simulink model "led_flash"  (R2023b)
settings: Solver=FixedStepAuto  StartTime=0.0  StopTime=999  RelTol=1e-3  EnableMultiTasking=on
libraries: mbedblockslib x11, raspberrypiIMUsensorslib x1, eeQuadratureDecoder x1
settings Model: ExtModeTrigDuration=10  Creator=Aidan  LastModifiedBy=Aidan
settings SolverCC: AutoInsertRateTranBlk=on
settings OptimizationCC: EnhancedBackFolding=on  PassReuseOutputArgsAs=Individual arguments  ZeroExternalMemoryAtStartup=off  ZeroInternalMemoryAtStartup=off  MaxStackSize=64  OptimizeBlockOrder=speed  DifferentSizesBufferReuse=on  OptimizationCustomize=off  EfficientTunableParamExpr=on
settings DebuggingCC: ParameterTunabilityLossMsg=error
settings HardwareCC: ProdBitPerPointer=32  ProdBitPerSizeT=32  ProdBitPerPtrDiffT=32  ProdLargestAtomicInteger=Long  ProdLargestAtomicFloat=Double  ProdWordSize=32  ProdLongLongMode=on  ProdHWDeviceType=ARM Compatible->ARM Cortex  UseEmbeddedCoderFeatures=off
settings SFSimCC: MATLABDynamicMemAlloc=off
settings RTWCC: Description=Embedded Coder  SystemTargetFile=ert.tlc  HardwareBoard=STM32 Nucleo F746ZG  TemplateMakefile=ert_default_tmf  Toolchain=GNU Tools for ARM Embedded Processors
settings CodeAppCC: ForceParamTrailComments=on  IgnoreCustomStorageClasses=off  OperatorAnnotations=on  SimulinkDataObjDesc=on  SFDataObjDesc=on  InsertBlockDesc=on
settings ERTTargetCC: SupportNonInlinedSFcns=on  ExtModeTransport=3  ExtModeStaticAlloc=on  ExtModeStaticAllocSize=2000  ExtModeMexFile=ext_xcp  ExtModeIntrfLevel=Level2 - Open

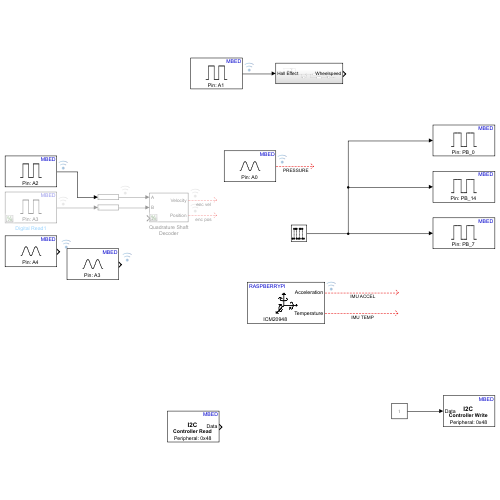
[thumbnail: Simulink's stored preview of the top-level diagram]
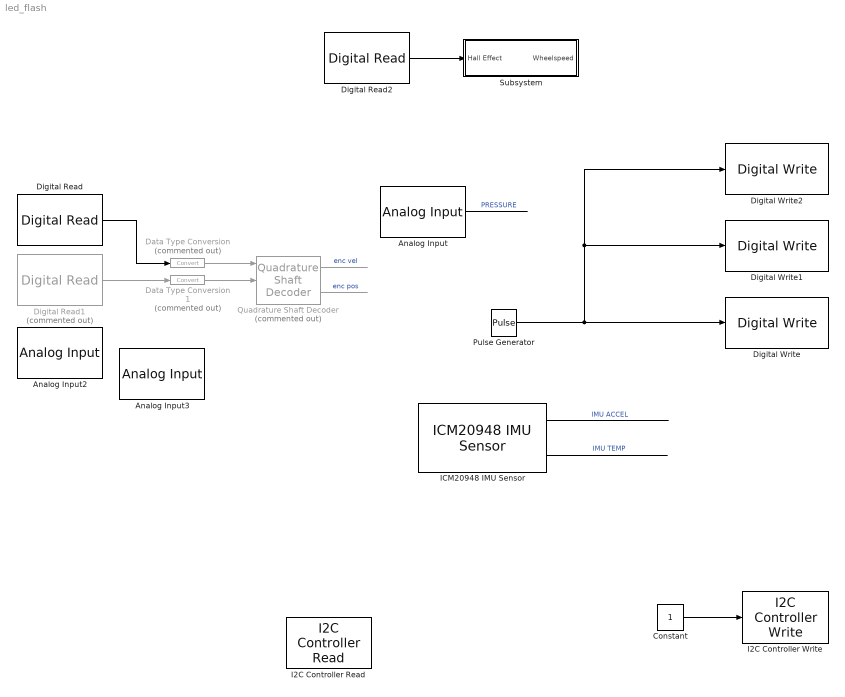
== system led_flash ==
  Analog Input : mbedblockslib/Analog Input  Pin=A0  ReadResultsOnly=off  ConversionTriggerSource=Software  ExternalTriggerType=uint32( 0 )  OutputDataType=double  EnableConversionCompleteNotify=off  EnableOuputStatus=off  SampleTime=-1
      settings: LibrarySourceBlock=stmnucleorootlib/Common/Analog Input
  Analog Input2 : mbedblockslib/Analog Input  Pin=A4  ReadResultsOnly=off  ConversionTriggerSource=Software  ExternalTriggerType=uint32( 0 )  OutputDataType=double  EnableConversionCompleteNotify=off  EnableOuputStatus=off  SampleTime=-1
      settings: LibrarySourceBlock=stmnucleorootlib/Common/Analog Input
  Analog Input3 : mbedblockslib/Analog Input  Pin=A3  ReadResultsOnly=off  ConversionTriggerSource=Software  ExternalTriggerType=uint32( 0 )  OutputDataType=double  EnableConversionCompleteNotify=off  EnableOuputStatus=off  SampleTime=-1
      settings: LibrarySourceBlock=stmnucleorootlib/Common/Analog Input
  Constant : Constant
  Data Type Conversion : DataTypeConversion  Commented=on  SaturateOnIntegerOverflow=off  RndMeth=Floor
  Data Type Conversion1 : DataTypeConversion  Commented=on  SaturateOnIntegerOverflow=off  RndMeth=Floor
  Digital Read : mbedblockslib/Digital Read  Pin=A2  Direction=input  SampleTime=-1
      settings: LibrarySourceBlock=stmnucleorootlib/Common/Digital Read
  Digital Read1 : mbedblockslib/Digital Read  Commented=on  Pin=A3  Direction=input  SampleTime=-1
      settings: LibrarySourceBlock=stmnucleorootlib/Common/Digital Read
  Digital Read2 : mbedblockslib/Digital Read  Pin=A1  Direction=input  SampleTime=-1
      settings: LibrarySourceBlock=stmnucleorootlib/Common/Digital Read
  Digital Write : mbedblockslib/Digital Write  Pin=PB_7  Direction=output
  Digital Write1 : mbedblockslib/Digital Write  Pin=PB_14  Direction=output
  Digital Write2 : mbedblockslib/Digital Write  Pin=PB_0  Direction=output
  I2C Controller Read : mbedblockslib/I2C Controller Read  I2CModule=0  Mode=Master  SlaveAddress=hex2dec('48')  SlaveByteOrder=BigEndian  Direction=Receiver  RegisterAddressMode=on  RegisterAddress=uint8(1)  SlaveDataType=uint8  DataLength=2  NoAck=off  RepeatedStart=off  OutputStatus=off  SampleTime=0.1
      settings: LibrarySourceBlock=stmnucleorootlib/Common/I2C Controller Read
  I2C Controller Write : mbedblockslib/I2C Controller Write  I2CModule=0  Mode=Master  SlaveAddress=hex2dec('48')  SlaveByteOrder=BigEndian  Direction=Transmitter  RegisterAddressMode=on  RegisterAddress=uint8(1)  SlaveDataType=uint8  DataLength=2  NoAck=off  RepeatedStart=off  OutputStatus=off
      settings: LibrarySourceBlock=stmnucleorootlib/Common/I2C Controller Write
  ICM20948 IMU Sensor : raspberrypiIMUsensorslib/ICM20948 IMU Sensor  I2CModule=0  I2CAddress=0x69  BitRate=1000000  EnableDRDY=off  InterruptType=Active high  IsActiveAccel=on  IsActiveGyro=off  IsActiveMag=off  IsActiveTemp=on  IsActiveStatus=off  IsActiveTimeStamp=off  AccelerometerRange=+/-2g  AccelerometerODR=1125  AccelerometerBW=23.9 Hz  GyroscopeRange=+/-250 dps  GyroscopeODR=1125  GyroscopeBW=23.9 Hz  MagnetometerODR=100 Hz  TemperatureBW=34.1 Hz  DataType=double  SampleTime=-1  QueueSizeFactor=3
  Pulse Generator : DiscretePulseGenerator  SampleTime=0.1
  Quadrature Shaft Decoder : eeQuadratureDecoder/Quadrature Shaft Decoder  Commented=on  NPulse=2048  Ts=-1
      settings: LibrarySourceBlock=|
      | ee_sl_lib/Observers/Quadrature Shaft
      | Decoder
  Subsystem : Subsystem
  wires:
  Pulse Generator/1 -> Digital Write/1, Digital Write1/1, Digital Write2/1
  ICM20948 IMU Sensor/1 -> ?  "IMU ACCEL"
  ICM20948 IMU Sensor/2 -> ?  "IMU TEMP"
  Analog Input/1 -> ?  "PRESSURE"
  Digital Read1/1 -> Data Type Conversion1/1
  Digital Read/1 -> Data Type Conversion/1
  Data Type Conversion/1 -> Quadrature Shaft Decoder/1
  Data Type Conversion1/1 -> Quadrature Shaft Decoder/2
  Quadrature Shaft Decoder/1 -> ?  "enc vel"
  Quadrature Shaft Decoder/2 -> ?  "enc pos"
  Digital Read2/1 -> Subsystem/1(Hall Effect)
  Constant/1 -> I2C Controller Write/1

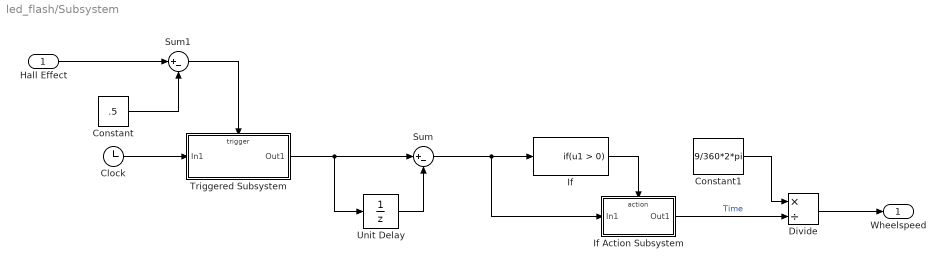
== system led_flash/Subsystem ==
  Hall Effect : Inport
  Clock : Clock
  Constant : Constant  Value=.5
  Constant1 : Constant  Value=9/360*2*pi
  Divide : Product  Inputs=*/
  If : If  ShowElse=off
  If Action Subsystem : Subsystem  TreatAsAtomicUnit=on
  Sum : Sum  Inputs=|+-
  Sum1 : Sum  Inputs=|+-
  Triggered Subsystem : Subsystem  TreatAsAtomicUnit=on
  Unit Delay : UnitDelay  SampleTime=-1  HasFrameUpgradeWarning=on
  Wheelspeed : Outport
  wires:
  Constant1/1 -> Divide/1
  Sum1/1 -> Triggered Subsystem/Trigger
  If Action Subsystem/1(Out1) -> Divide/2  "Time"
  If/1 -> If Action Subsystem/Action
  Sum/1 -> If Action Subsystem/1(In1), If/1
  Hall Effect/1 -> Sum1/1
  Clock/1 -> Triggered Subsystem/1(In1)
  Unit Delay/1 -> Sum/2
  Triggered Subsystem/1(Out1) -> Sum/1, Unit Delay/1
  Constant/1 -> Sum1/2
  Divide/1 -> Wheelspeed/1

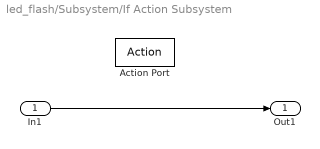
== system led_flash/Subsystem/If Action Subsystem ==
  In1 : Inport
  Action Port : ActionPort  ActionPortLabel=if(u1 > 0)
  Out1 : Outport
  wires:
  In1/1 -> Out1/1

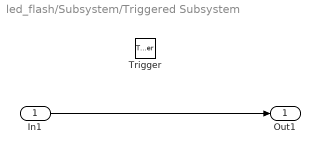
== system led_flash/Subsystem/Triggered Subsystem ==
  In1 : Inport
  Trigger : TriggerPort  VariantControl=(inherit)
  Out1 : Outport
  wires:
  In1/1 -> Out1/1
